simulink model "exp5_10"  (Simulink 3.00)
settings: Solver=ode45  SolverMode=SingleTasking  StartTime=0.0  StopTime=10.0  RelTol=1e-3  AbsTol=1e-6
settings Model: TimeSaveName=t  OutputSaveName=y  FinalStateName=yy  RTWTemplateMakefile=grt_vc.tmf

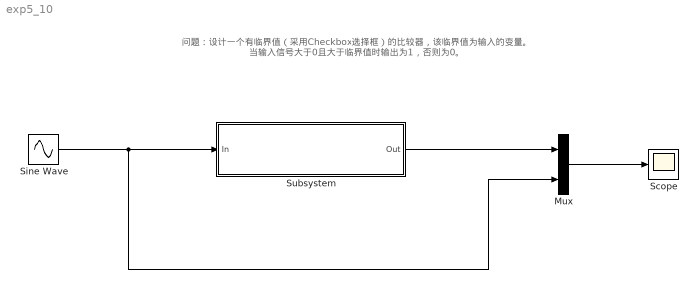
== system exp5_10 ==
  note: 问题：设计一个有临界值（采用Checkbox选择框）的比较器，该临界值为输入的变量。
      | 当输入信号大于0且大于临界值时输出为1，否则为0。
  Mux : Mux  Inputs=2
  Scope : Scope
      settings: TickLabels=on  TimeRange=10  YMin=-2  YMax=2  SaveToWorkspace=off  SaveName=ScopeData  DataFormat=Matrix
  Sine Wave : Sin  Amplitude=1  Frequency=1  Phase=0  SampleTime=0
  Subsystem : Subsystem  mask(comparater){t=on}
      mask prompts: t "threshold on"
      mask help: The block will translate the input signal to square wave. If the checkbox 'threshold on' is selected then threshold is 0.5, otherwise, there is no threshold.
      mask init:
      | if t
      | th=0.5;
      | else
      | th=0;
      | end
      mask Help: Select the checkbox 'threshold on' to access the threshold function.
      mask Display: disp('The Comparater')
  wires:
  Subsystem/1(Out) -> Mux/1
  Mux/1 -> Scope/1
  Sine Wave/1 -> Subsystem/1(In), Mux/2

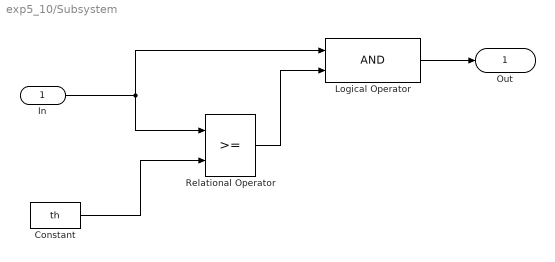
== system exp5_10/Subsystem ==
  In : Inport  Port=1  PortWidth=-1  SampleTime=-1  DataType=auto
      settings: SignalType=auto
  Constant : Constant  Value=th
  Logical Operator : Logic  Operator=AND  Inputs=2
  Relational Operator : RelationalOperator  Operator=>=
  Out : Outport  Port=1  InitialOutput=0
  wires:
  Relational Operator/1 -> Logical Operator/2
  Constant/1 -> Relational Operator/2
  In/1 -> Relational Operator/1, Logical Operator/1
  Logical Operator/1 -> Out/1
